simulink library "Lib_Rev2_Dvcu_Anlg"  (R2019b)
settings: Solver=ode45  StartTime=0.0  StopTime=10.0  RelTol=1e-3  EnableMultiTasking=on
settings Model: Creator=kmansour  LastModifiedBy=depl_
settings DataIOCC: LimitDataPoints=on  SaveFormat=Array  ReturnWorkspaceOutputs=off
settings OptimizationCC: LifeSpan=inf
settings DebuggingCC: AllowSymbolicDim=off  SFUnexpectedBacktrackingDiag=warning  SFNoUnconditionalDefaultTransitionDiag=warning  SFExecutionAtInitializationDiag=none  ArithmeticOperatorsInVariantConditions=warning
settings HardwareCC: ProdBitPerPointer=32  ProdBitPerSizeT=32  ProdBitPerPtrDiffT=32  ProdLargestAtomicFloat=None  ProdIntDivRoundTo=Undefined  ProdEndianess=Unspecified  ProdWordSize=32  ProdHWDeviceType=32-bit Generic
settings ModelReferenceCC: PropagateSignalLabelsOutOfModel=off
settings SFSimCC: SimUseLocalCustomCode=off  CustomCodeUndefinedFunction=UseInterfaceOnly
settings RTWCC: RTWUseLocalCustomCode=off
settings CodeAppCC: StateflowObjectComments=on
settings GRTTargetCC: TargetLangStandard=C89/C90 (ANSI)  GeneratePreprocessorConditionals=Disable all
settings ConfigComp: CovMetricSettings=dw  CovHtmlReporting=on  CovSaveCumulativeToWorkspaceVar=on  CovSaveSingleToWorkspaceVar=on  CovExternalEMLEnable=off

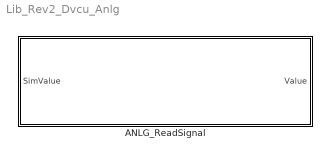
== system Lib_Rev2_Dvcu_Anlg ==
  ANLG_ReadSignal : Subsystem  TreatAsAtomicUnit=on  mask{PARAM_ID=ECU_ANLG_ADC_5V_P60}
      mask prompts: PARAM_ID "Choose a Signal"
      mask TypeOptions PARAM_ID: ECU_ANLG_ADC_5V_P60 | ECU_ANLG_ADC_5V_P30 | ECU_ANLG_ADC_5V_P29 | ECU_ANLG_ADC_5V_P69 | ECU_ANLG_ADC_5V_P59 | ECU_ANLG_ADC_5V_P49 | ECU_ANLG_ADC_5V_P50 | ECU_ANLG_POWER_SUPPLY24V | ECU_ANLG_ADC_5V_P39 | ECU_ANLG_ADC_5V_P40 | ECU_ANLG_ADC_5V_P73 | ECU_ANLG_ADC_5V_P75 | ECU_ANLG_ADC_5V_P74 | ECU_ANLG_ADC_5V_P72 | ECU_ANLG_ADC_5V_P71 | ECU_ANLG_ADC_5V_P80 | ECU_ANLG_ADC_5V_P79 | ECU_ANLG_ADC_5V_P78 | ECU_ANLG_ADC_5V_P77 | ECU_ANLG_ADC_5V_P76 | ECU_ANLG_ADC_5V_P70 | ECU_ANLG_TEMP_SENSOR1 | ECU_ANLG_TEMP_SENSOR2
      mask Display:
      | image(imread('devcu_final.png'),'top-left');
      | color('black');
      | port_label('input', 1, 'SimValue');
      | port_label('output', 1, 'Value');
      | 
      | strCell =get_param(gcb, 'MaskValues');
      | strCell = strtrim(strCell);
      | str = strCell{1};
      | str = strrep(str, '_', '\_');
      | disp(str, 'texmode', 'on');

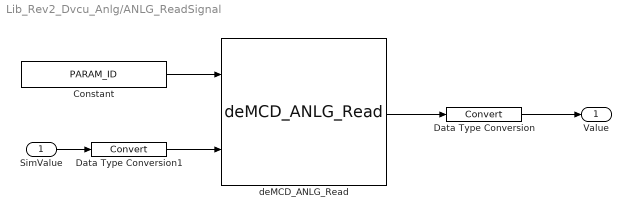
== system Lib_Rev2_Dvcu_Anlg/ANLG_ReadSignal ==
  SimValue : Inport
  Constant : Constant  Value=PARAM_ID
  Data Type Conversion : DataTypeConversion
  Data Type Conversion1 : DataTypeConversion
  deMCD_ANLG_Read : S-Function  FunctionName=deMCD_ANLG_Read  SFunctionDeploymentMode=off  EnableBusSupport=off
      mask Display:
      | image(imread('logo_deMCD_white_background.png'),'center');
      | color('black');
      | port_label('input', 1, 'ID');
      | port_label('input', 2, 'SimValue');
      | port_label('output', 1, 'Value');
  Value : Outport
  wires:
  deMCD_ANLG_Read/1 -> Data Type Conversion/1
  Constant/1 -> deMCD_ANLG_Read/1
  Data Type Conversion/1 -> Value/1
  Data Type Conversion1/1 -> deMCD_ANLG_Read/2
  SimValue/1 -> Data Type Conversion1/1
